simulink model "Three_phase_full_wave_full_controlled_rectifier"  (R2022b)
settings: Solver=ode23tb  StartTime=0.0  StopTime=0.5  RelTol=1e-3
libraries: spsThyristorLib x6, spsACVoltageSourceLib x3, spsMultimeterLib x2, spsGroundLib x1, spsMeanLib x1, spsSeriesRLCBranchLib x1, spsVoltageMeasurementLib x1, sps_lib x1
settings Model: Creator=Biplov Jha  LastModifiedBy=Biplov Jha

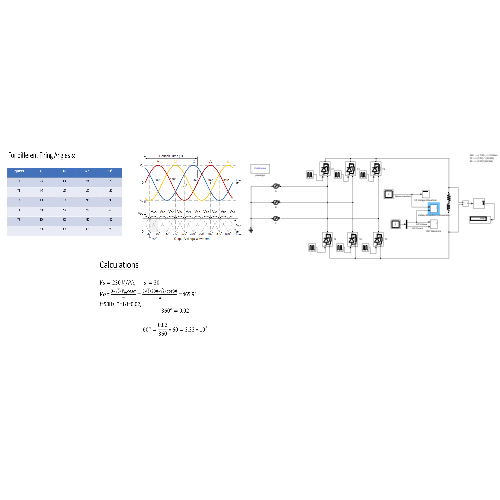
[thumbnail: Simulink's stored preview of the top-level diagram]
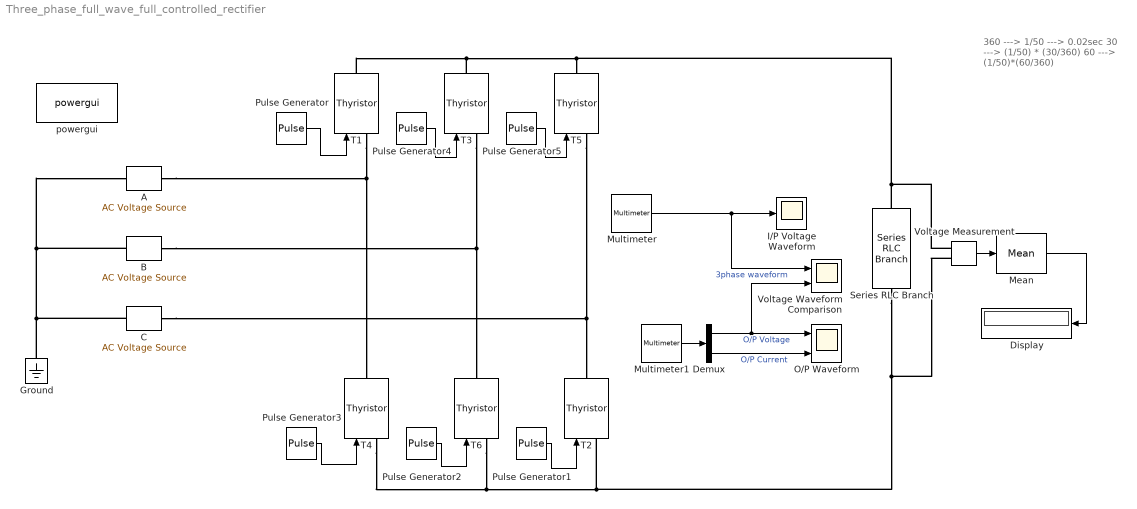
== system Three_phase_full_wave_full_controlled_rectifier ==
  note: 360   ---> 1/50 ---> 0.02sec
      | 30 ---> (1/50) * (30/360)
      | 60 ---> (1/50)*(60/360)
  A : spsACVoltageSourceLib/AC Voltage Source  Amplitude=230*sqrt(2)  Phase=0  Frequency=50  SampleTime=0  Measurements=Voltage  BusType=swing  Pref=10e3  Qref=0  Qmin=-inf  Qmax=+inf
  B : spsACVoltageSourceLib/AC Voltage Source  Amplitude=230*sqrt(2)  Phase=120  Frequency=50  SampleTime=0  Measurements=Voltage  BusType=swing  Pref=10e3  Qref=0  Qmin=-inf  Qmax=+inf
  C : spsACVoltageSourceLib/AC Voltage Source  Amplitude=230*sqrt(2)  Phase=-120  Frequency=50  SampleTime=0  Measurements=Voltage  BusType=swing  Pref=10e3  Qref=0  Qmin=-inf  Qmax=+inf
  Demux : Demux  Outputs=2
  Display : Display
  Ground : spsGroundLib/Ground  LConnTagsString=a
  I/P Voltage Waveform : Scope
  Mean : spsMeanLib/Mean  Freq=60  Vinit=0  Ts=0
  Multimeter : spsMultimeterLib/Multimeter  L=5  sel=[2 3 4]  yselected={}  Gain=[1 1 1]  OutputType=Complex  PlotAtSimulationStop=off  PhasorSimulation=off
  Multimeter1 : spsMultimeterLib/Multimeter  L=5  sel=[1 5]  yselected={}  Gain=[1 1]  OutputType=Complex  PlotAtSimulationStop=off  PhasorSimulation=off
  O/P Waveform : Scope  NumInputPorts=2
  Pulse Generator : DiscretePulseGenerator  PulseType=Time based  Period=1/50  PulseWidth=(120/360)*100  PhaseDelay=(1/50)*(60/360)
  Pulse Generator1 : DiscretePulseGenerator  PulseType=Time based  Period=1/50  PulseWidth=(120/360)*100  PhaseDelay=(1/50)*(120/360)
  Pulse Generator2 : DiscretePulseGenerator  PulseType=Time based  Period=1/50  PulseWidth=(120/360)*100  PhaseDelay=(1/50)*(360/360)
  Pulse Generator3 : DiscretePulseGenerator  PulseType=Time based  Period=1/50  PulseWidth=(120/360)*100  PhaseDelay=(1/50)*(240/360)
  Pulse Generator4 : DiscretePulseGenerator  PulseType=Time based  Period=1/50  PulseWidth=(120/360)*100  PhaseDelay=(1/50)*(180/360)
  Pulse Generator5 : DiscretePulseGenerator  PulseType=Time based  Period=1/50  PulseWidth=(120/360)*100  PhaseDelay=(1/50)*(300/360)
  Series RLC Branch : spsSeriesRLCBranchLib/Series RLC Branch  LConnTagsString=__new0  RConnTagsString=__new0  BranchType=RL  Resistance=5  Inductance=650e-3  SetiL0=off  InitialCurrent=0  Capacitance=1e-6  Setx0=off  InitialVoltage=0  Measurements=Branch voltage and current
  T{1..6} (6 alike) : spsThyristorLib/Thyristor  Ron=0.001  Lon=0  Vf=0.8  IC=0  Rs=500  Cs=250e-9  Measurements=off
  Voltage Measurement : spsVoltageMeasurementLib/Voltage Measurement  PhasorSimulation=off  OutputType=Complex  PSBequivalent=0
  Voltage Waveform Comparison : Scope  NumInputPorts=2
  powergui : sps_lib/powergui  Priority=1  SimulationMode=Continuous  SampleTime=50e-6  frequency=60  Iterations=50  frequencyindice=50  Pbase=100e6  ErrMax=1e-4  UnitsV=kV  UnitsW=MW  buscounter=0  FunctionMessages=off  echomessages=off  EnableUseOfTLC=off  CurrentSourceSwitches=off  DisableSnubberDevices=off  DisableRonSwitches=off  DisableVfSwitches=off  DisplayEquations=off  AutomaticDiscreteSolvers=off  SolverType=Tustin/Backward Euler (TBE)  Interpol=off  ExternalGateDelay=off  methode=off  Ts=100  x0status=blocks  SPID=on  SwTol=0  HookPort=off  NonlinearTolerance=1e-4  nMaxIteration=100  ContinueOnMaxIteration=off  RestoreLinks=warning  ResistiveCurrentMeasurement=off  Frange=[0:2:500]  Ylog=off  Xlog=on  ShowGrid=off  save=off  variable=ZData  structure=0  ZoomFFT=off  StartTime=0.0  cycles=1  DisplayStyle=1  fundamental=60  FreqAxis=off  MaxFrequency=1000  frequencyindicesteady=1  RmsSteady=1  display=off
  wires:
  Multimeter/1 -> I/P Voltage Waveform/1, Voltage Waveform Comparison/1  "3phase waveform"
  Multimeter1/1 -> Demux/1
  Demux/1 -> O/P Waveform/1, Voltage Waveform Comparison/2  "O/P Voltage"
  Demux/2 -> O/P Waveform/2  "O/P Current"
  Pulse Generator/1 -> T1/1
  Pulse Generator4/1 -> T3/1
  Pulse Generator5/1 -> T5/1
  Pulse Generator1/1 -> T2/1
  Pulse Generator2/1 -> T6/1
  Pulse Generator3/1 -> T4/1
  Voltage Measurement/1 -> Mean/1
  Mean/1 -> Display/1
  connections:
  Ground/LConn1 -- C/LConn1 -- B/LConn1 -- A/LConn1
  T1/RConn1 -- T3/RConn1 -- Voltage Measurement/LConn1 -- Series RLC Branch/LConn1 -- T5/RConn1
  T4/LConn1 -- T6/LConn1 -- Voltage Measurement/LConn2 -- Series RLC Branch/RConn1 -- T2/LConn1
  T1/LConn1 -- A/RConn1 -- T4/RConn1
  T3/LConn1 -- B/RConn1 -- T6/RConn1
  T5/LConn1 -- T2/RConn1 -- C/RConn1
